simulink model "Copy_of_battery"  (R2021a)
settings: Solver=ode3  StartTime=0.0  StopTime=inf  FixedStep=T_est  RelTol=1e-3  EnableMultiTasking=on
values from neighbouring files (symbols this model uses):
  drive_profile = [0.003069801 0.003247245 0.003020715 0.003053892 0.002820143 0.003317081 0.003158873 0.002919445 0.002956375 0.002698265 0.002861501 0.002770798 ... (18750 elements, 1x18750)]    [drive_profile_ftp.mat]    (also in workspace.mat = [0 0 0 0 0 0 0 0 0 0 0 0 ... (521 elements, 1x521)]; workspace_2rc.mat; workspace_comparison.mat)
  drive_profile_index = [1 2 3 4 5 6 7 8 9 10 11 12 ... (18750 elements, 1x18750)]    [drive_profile_ftp.mat]    (also in load_sim_data_v2.m = drive_profile_index - 1; workspace.mat = [0 0.115384615385 0.230769230769 0.346153846154 0.4615384615; workspace_2rc.mat; workspace_comparison.mat)
  initial_soc = interp1(voc_soc_lut, voc_soc_lut_index, initial_vterm)    [load_sim_data.m]    (also in load_sim_data_v2.m)
  Q_total = 236.8    [load_sim_data.m]    (also in load_sim_data_v2.m = 350; workspace.mat = 44; workspace_2rc.mat = 44; workspace_comparison.mat = 44)
  R1 = interp2(temp_array, voc_array, R1_array, initial_temp, initial_voc)    [load_sim_data.m]    (also in load_sim_data_v2.m; workspace.mat = 0.00033425; workspace_2rc.mat = 0.0001483; workspace_comparison.mat = 0.0001483)
  R2 = interp2(temp_array, voc_array, R2_array, initial_temp, initial_voc)    [load_sim_data.m]    (also in load_sim_data_v2.m; workspace.mat = 0.000915125; workspace_2rc.mat = 0.0001594; workspace_comparison.mat = 0.0001594)
  Ri = interp2(temp_array, voc_array, Ri_array, initial_temp, initial_voc)    [load_sim_data.m]    (also in load_sim_data_v2.m; workspace.mat = 0.000736040625; workspace_2rc.mat = 0.0007932; workspace_comparison.mat = 0.0007932)
  sim_time = drive_profile_index(end)    [load_sim_data.m]    (also in load_sim_data_v2.m)
  voc_soc_lut = [3.07420931 3.44278771 3.51037487 3.58546258 3.63776945 3.68066188 3.73931818 3.84140797 3.94332291 4.0535654 4.18301283]    [emf_curve_single.mat]    (also in workspace.mat = [2.9985 3.0047 3.1504 3.2397 3.3026 3.3438 3.3699 3.3878 3.4; workspace_2rc.mat = [2.9985 3.0047 3.1504 3.2397 3.3026 3.3438 3.3699 3.3878 3.4; workspace_comparison.mat = [2.9985 3.0047 3.1504 3.2397 3.3026 3.3438 3.3699 3.3878 3.4)
  voc_soc_lut_index = [0 10 20 30 40 50 60 70 80 90 100]    [emf_curve_single.mat]    (also in workspace.mat = [0 1.6393442623 3.27868852459 4.91803278689 6.55737704918 8.; workspace_2rc.mat = [0 1.6393442623 3.27868852459 4.91803278689 6.55737704918 8.; workspace_comparison.mat = [0 1.6393442623 3.27868852459 4.91803278689 6.55737704918 8.)
libraries: fl_lib x17, nesl_utility x11
settings Model: Creator=OTG00077  LastModifiedBy=avramkachura
settings SolverCC: AlgebraicLoopSolver=TrustRegion
settings DataIOCC: LimitDataPoints=on  SaveFormat=Array  ReturnWorkspaceOutputs=off
settings OptimizationCC: LifeSpan=inf
settings DebuggingCC: SolverPrmCheckMsg=warning  SFUnexpectedBacktrackingDiag=warning  SFNoUnconditionalDefaultTransitionDiag=warning  SFExecutionAtInitializationDiag=none  SFMachineParentedDataDiag=warning  ArithmeticOperatorsInVariantConditions=warning
settings HardwareCC: ProdBitPerPointer=32  ProdBitPerSizeT=32  ProdBitPerPtrDiffT=32  ProdLargestAtomicFloat=None  ProdIntDivRoundTo=Undefined  ProdEndianess=Unspecified  ProdWordSize=32  ProdHWDeviceType=32-bit Generic
settings ModelReferenceCC: PropagateSignalLabelsOutOfModel=off
settings SFSimCC: SimUseLocalCustomCode=off  CustomCodeUndefinedFunction=UseInterfaceOnly
settings RTWCC: RTWUseLocalCustomCode=off
settings CodeAppCC: StateflowObjectComments=on
settings GRTTargetCC: TargetLangStandard=C89/C90 (ANSI)
settings ConfigComp: CovMetricSettings=dw  CovSaveCumulativeToWorkspaceVar=on  CovSaveSingleToWorkspaceVar=on  CovExternalEMLEnable=off  CovSFcnEnable=off
settings SimscapeCC: SimscapeNormalizeSystem=off

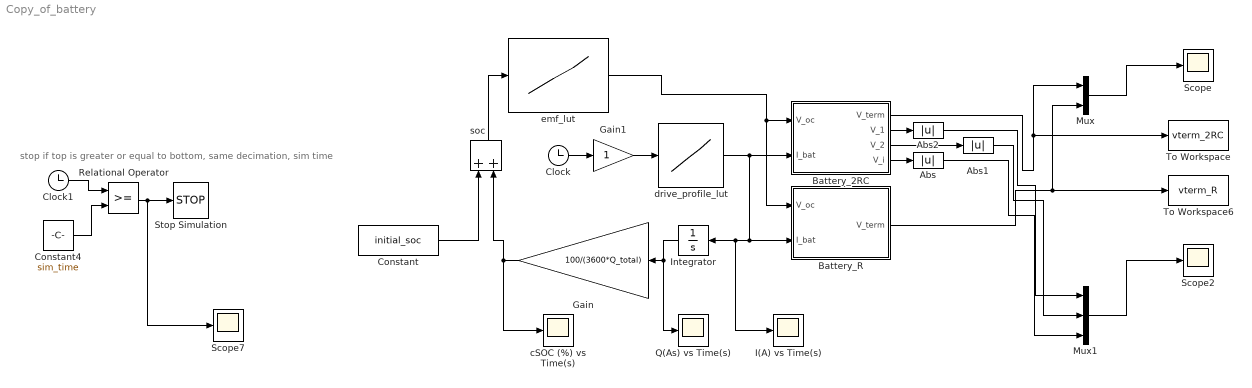
== system Copy_of_battery ==
  note: stop if top is greater or equal to bottom, same decimation, sim time
  Abs : Abs
  Abs1 : Abs
  Abs2 : Abs
  Battery_2RC : Subsystem
  Battery_R : Subsystem
  Clock : Clock
      settings: Decimation=100
  Clock1 : Clock
      settings: Decimation=100
  Constant : Constant  Value=initial_soc
  Constant4 : Constant  Value=sim_time
  Gain : Gain  Gain=100/(3600*Q_total)
  Gain1 : Gain
  I(A) vs Time(s) : Scope
  Integrator : Integrator
  Mux : Mux  Inputs=2
  Mux1 : Mux  Inputs=3
  Q(As) vs Time(s) : Scope
  Relational Operator : RelationalOperator  OutDataTypeStr=boolean  RndMeth=Simplest
  Scope : Scope
  Scope2 : Scope
  Scope7 : Scope
  Stop Simulation : Stop
  To Workspace : ToWorkspace  VariableName=vterm_2RC  SampleTime=-1
      settings: Decimation=100
  To Workspace6 : ToWorkspace  VariableName=vterm_R  SampleTime=-1
      settings: Decimation=100
  "cSOC (%) vs Time(s) " : Scope
  drive_profile_lut : Lookup_n-D  NumberOfTableDimensions=1  BreakpointsForDimension1=drive_profile_index  Table=drive_profile  InternalRulePriority=Speed  RndMeth=Simplest  InputSameDT=on
  emf_lut : Lookup_n-D  NumberOfTableDimensions=1  BreakpointsForDimension1=voc_soc_lut_index  Table=voc_soc_lut  InternalRulePriority=Speed  RndMeth=Simplest  InputSameDT=on
  soc : Sum
  wires:
  Integrator/1 -> Q(As) vs Time(s)/1, Gain/1
  Gain/1 -> "cSOC (%) vs Time(s) "/1, soc/2
  soc/1 -> emf_lut/1
  Constant/1 -> soc/1
  emf_lut/1 -> Battery_R/1(V_oc), Battery_2RC/1(V_oc)
  drive_profile_lut/1 -> Battery_2RC/2(I_bat), I(A) vs Time(s)/1, Integrator/1, Battery_R/2(I_bat)
  Battery_2RC/1(V_term) -> Mux/1, To Workspace/1
  Clock/1 -> Gain1/1
  Gain1/1 -> drive_profile_lut/1
  Mux/1 -> Scope/1
  Battery_R/1(V_term) -> Mux/2, To Workspace6/1
  Battery_2RC/4(V_i) -> Abs/1
  Battery_2RC/3(V_2) -> Abs1/1
  Battery_2RC/2(V_1) -> Abs2/1
  Abs2/1 -> Mux1/1
  Abs1/1 -> Mux1/2
  Abs/1 -> Mux1/3
  Mux1/1 -> Scope2/1
  Relational Operator/1 -> Scope7/1, Stop Simulation/1
  Constant4/1 -> Relational Operator/2
  Clock1/1 -> Relational Operator/1

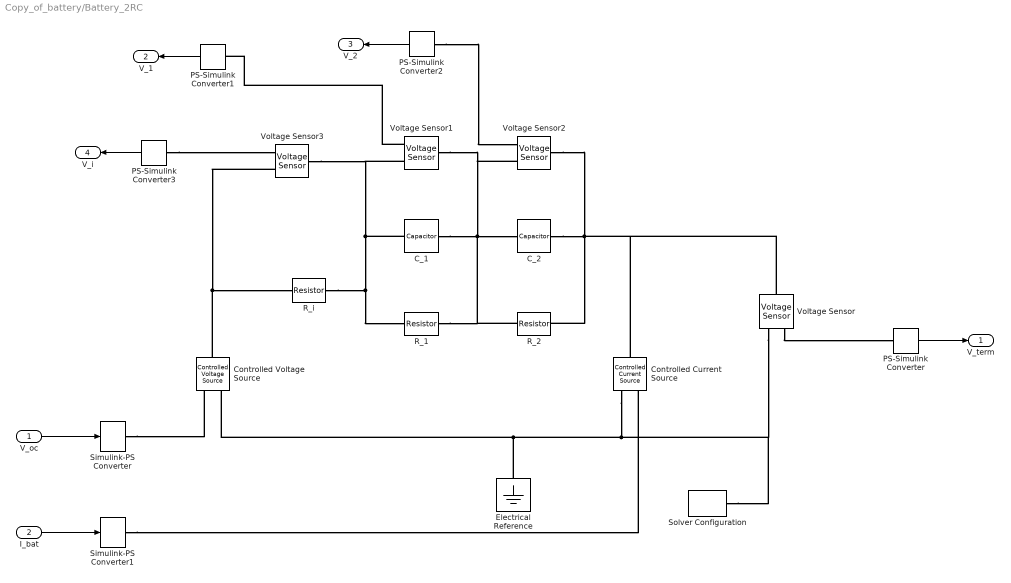
== system Copy_of_battery/Battery_2RC ==
  V_oc : Inport
  I_bat : Inport  Port=2
  C_1 : fl_lib/Electrical/Electrical Elements/Capacitor  c=C1 F  r=0 Ohm  g=0 1/Ohm  i_specify=off  i_priority=High  i=0 A  i_nominal_specify=off  i_nominal_unit=A  i_nominal_value=1  v_specify=off  v_priority=High  v=0 V  v_nominal_specify=off  v_nominal_unit=V  v_nominal_value=1  vc_specify=off  vc_priority=High  vc=0 V  vc_nominal_specify=off  vc_nominal_unit=V  vc_nominal_value=1
  C_2 : fl_lib/Electrical/Electrical Elements/Capacitor  c=C2 F  r=0 Ohm  g=0 1/Ohm  i_specify=off  i_priority=High  i=0 A  i_nominal_specify=off  i_nominal_unit=A  i_nominal_value=1  v_specify=off  v_priority=High  v=0 V  v_nominal_specify=off  v_nominal_unit=V  v_nominal_value=1  vc_specify=off  vc_priority=High  vc=0 V  vc_nominal_specify=off  vc_nominal_unit=V  vc_nominal_value=1
  Controlled Current Source : fl_lib/Electrical/Electrical Sources/Controlled Current Source
  Controlled Voltage Source : fl_lib/Electrical/Electrical Sources/Controlled Voltage Source
  Electrical Reference : fl_lib/Electrical/Electrical Elements/Electrical Reference
  PS-Simulink Converter{,1..3} (4 alike) : nesl_utility/PS-Simulink Converter  PhysicalDomain=network_engine_domain  SubClassName=ps_output  LeftPortType=input  RightPortType=output  PseudoPeriodic=off  Frequencies=[]  Unit=1  AffineConversion=off
      settings: SourceProductBaseCode=PW,SS
  R_1 : fl_lib/Electrical/Electrical Elements/Resistor  R=R1 Ohm  i_specify=off  i_priority=High  i=0 A  i_nominal_specify=off  i_nominal_unit=A  i_nominal_value=1  v_specify=off  v_priority=High  v=0 V  v_nominal_specify=off  v_nominal_unit=V  v_nominal_value=1
  R_2 : fl_lib/Electrical/Electrical Elements/Resistor  R=R2 Ohm  i_specify=off  i_priority=High  i=0 A  i_nominal_specify=off  i_nominal_unit=A  i_nominal_value=1  v_specify=off  v_priority=High  v=0 V  v_nominal_specify=off  v_nominal_unit=V  v_nominal_value=1
  R_i : fl_lib/Electrical/Electrical Elements/Resistor  R=Ri Ohm  i_specify=off  i_priority=High  i=0 A  i_nominal_specify=off  i_nominal_unit=A  i_nominal_value=1  v_specify=off  v_priority=High  v=0 V  v_nominal_specify=off  v_nominal_unit=V  v_nominal_value=1
  Simulink-PS Converter : nesl_utility/Simulink-PS Converter  PhysicalDomain=network_engine_domain  SubClassName=ps_input  LeftPortType=input  RightPortType=output  PseudoPeriodic=off  Frequencies=[]  NoiseDistribution=none  NoiseParameters=[]  Unit=1  AffineConversion=off  FilteringAndDerivatives=zero  SimscapeFilterOrder=1  InputFilterTimeConstant=0.001  UdotUserProvided=1
      settings: SourceProductBaseCode=PW,SS
  Simulink-PS Converter1 : nesl_utility/Simulink-PS Converter  PhysicalDomain=network_engine_domain  SubClassName=ps_input  LeftPortType=input  RightPortType=output  PseudoPeriodic=off  Frequencies=[]  NoiseDistribution=none  NoiseParameters=[]  Unit=1  AffineConversion=off  FilteringAndDerivatives=zero  SimscapeFilterOrder=1  InputFilterTimeConstant=0.001  UdotUserProvided=1
      settings: SourceProductBaseCode=PW,SS
  Solver Configuration : nesl_utility/Solver Configuration  PhysicalDomain=network_engine_domain  SubClassName=solver  LeftPortType=input  RightPortType=generic  Tones=[]  Harmonics=[]  SimulateNoise=off  Profile=off  UseLocalSampling=off  EnableSwitchedLinearOptims=on  FrequencyDomain=off  UseCCode=off  RelTol=0.001  AbsTol=1e-06  MinStep=1e-09  ToWorkspace=off  RevertToSquareIcSolve=off  NumHomotopyIterations=100  PhasorMode=off  PhasorModeNumHarmonics=1  DoDC=off  ResidualTolerance=1e-09  UseLocalSolver=off  LocalSolverChoice=NE_BACKWARD_EULER_ADVANCER  LocalSolverSampleTime=0.001  DoFixedCost=off  MaxNonlinIter=3  MaxModeIter=2  ComputeImpulses=off  ImpulseIterations=2  LinearAlgebra=Sparse  EquationFormulation=NE_TIME_EF  DelaysMemoryBudget=1024  AutomaticFiltering=on  FilteringTimeConstant=0.001  PartitionStorageMethod=AS_NEEDED  PartitionMemoryBudget=1024  PartitionMethod=FAST
      settings: SourceProductBaseCode=PW,SS
  Voltage Sensor{,1..3} (4 alike) : fl_lib/Electrical/Electrical Sensors/Voltage Sensor
  V_term : Outport  VectorParamsAs1DForOutWhenUnconnected=off
  V_1 : Outport  Port=2  VectorParamsAs1DForOutWhenUnconnected=off
  V_2 : Outport  Port=3  VectorParamsAs1DForOutWhenUnconnected=off
  V_i : Outport  Port=4  VectorParamsAs1DForOutWhenUnconnected=off
  wires:
  V_oc/1 -> Simulink-PS Converter/1
  PS-Simulink Converter/1 -> V_term/1
  I_bat/1 -> Simulink-PS Converter1/1
  PS-Simulink Converter1/1 -> V_1/1
  PS-Simulink Converter2/1 -> V_2/1
  PS-Simulink Converter3/1 -> V_i/1
  connections:
  R_i/RConn1 -- Voltage Sensor3/LConn1 -- Voltage Sensor1/RConn2 -- C_1/LConn1 -- R_1/LConn1
  C_1/RConn1 -- Voltage Sensor2/RConn2 -- Voltage Sensor1/LConn1 -- R_2/LConn1 -- R_1/RConn1 -- C_2/LConn1
  C_2/RConn1 -- Voltage Sensor2/LConn1 -- R_2/RConn1 -- Controlled Current Source/LConn1 -- Voltage Sensor/LConn1
  Controlled Voltage Source/LConn1 -- Voltage Sensor3/RConn2 -- R_i/LConn1
  Simulink-PS Converter/RConn1 -- Controlled Voltage Source/RConn1
  Voltage Sensor/RConn1 -- PS-Simulink Converter/LConn1
  Controlled Current Source/RConn2 -- Solver Configuration/RConn1 -- Voltage Sensor/RConn2 -- Electrical Reference/LConn1 -- Controlled Voltage Source/RConn2
  Simulink-PS Converter1/RConn1 -- Controlled Current Source/RConn1
  Voltage Sensor1/RConn1 -- PS-Simulink Converter1/LConn1
  PS-Simulink Converter2/LConn1 -- Voltage Sensor2/RConn1
  PS-Simulink Converter3/LConn1 -- Voltage Sensor3/RConn1

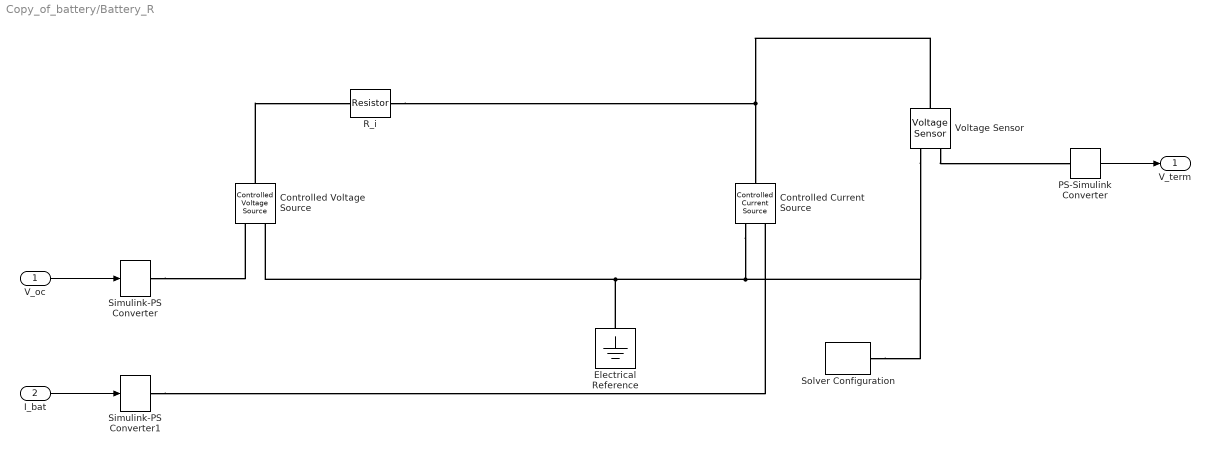
== system Copy_of_battery/Battery_R ==
  V_oc : Inport
  I_bat : Inport  Port=2
  Controlled Current Source : fl_lib/Electrical/Electrical Sources/Controlled Current Source
  Controlled Voltage Source : fl_lib/Electrical/Electrical Sources/Controlled Voltage Source
  Electrical Reference : fl_lib/Electrical/Electrical Elements/Electrical Reference
  PS-Simulink Converter : nesl_utility/PS-Simulink Converter  PhysicalDomain=network_engine_domain  SubClassName=ps_output  LeftPortType=input  RightPortType=output  PseudoPeriodic=off  Frequencies=[]  Unit=1  AffineConversion=off
      settings: SourceProductBaseCode=PW,SS
  R_i : fl_lib/Electrical/Electrical Elements/Resistor  R=Ri+R1+R2 Ohm  i_specify=off  i_priority=High  i=0 A  i_nominal_specify=off  i_nominal_unit=A  i_nominal_value=1  v_specify=off  v_priority=High  v=0 V  v_nominal_specify=off  v_nominal_unit=V  v_nominal_value=1
  Simulink-PS Converter : nesl_utility/Simulink-PS Converter  PhysicalDomain=network_engine_domain  SubClassName=ps_input  LeftPortType=input  RightPortType=output  PseudoPeriodic=off  Frequencies=[]  NoiseDistribution=none  NoiseParameters=[]  Unit=1  AffineConversion=off  FilteringAndDerivatives=zero  SimscapeFilterOrder=1  InputFilterTimeConstant=0.001  UdotUserProvided=1
      settings: SourceProductBaseCode=PW,SS
  Simulink-PS Converter1 : nesl_utility/Simulink-PS Converter  PhysicalDomain=network_engine_domain  SubClassName=ps_input  LeftPortType=input  RightPortType=output  PseudoPeriodic=off  Frequencies=[]  NoiseDistribution=none  NoiseParameters=[]  Unit=1  AffineConversion=off  FilteringAndDerivatives=zero  SimscapeFilterOrder=1  InputFilterTimeConstant=0.001  UdotUserProvided=1
      settings: SourceProductBaseCode=PW,SS
  Solver Configuration : nesl_utility/Solver Configuration  PhysicalDomain=network_engine_domain  SubClassName=solver  LeftPortType=input  RightPortType=generic  Tones=[]  Harmonics=[]  SimulateNoise=off  Profile=off  UseLocalSampling=off  EnableSwitchedLinearOptims=on  FrequencyDomain=off  UseCCode=off  RelTol=0.001  AbsTol=1e-06  MinStep=1e-09  ToWorkspace=off  RevertToSquareIcSolve=off  NumHomotopyIterations=100  PhasorMode=off  PhasorModeNumHarmonics=1  DoDC=off  ResidualTolerance=1e-09  UseLocalSolver=off  LocalSolverChoice=NE_BACKWARD_EULER_ADVANCER  LocalSolverSampleTime=0.001  DoFixedCost=off  MaxNonlinIter=3  MaxModeIter=2  ComputeImpulses=off  ImpulseIterations=2  LinearAlgebra=Sparse  EquationFormulation=NE_TIME_EF  DelaysMemoryBudget=1024  AutomaticFiltering=on  FilteringTimeConstant=0.001  PartitionStorageMethod=AS_NEEDED  PartitionMemoryBudget=1024  PartitionMethod=FAST
      settings: SourceProductBaseCode=PW,SS
  Voltage Sensor : fl_lib/Electrical/Electrical Sensors/Voltage Sensor
  V_term : Outport  VectorParamsAs1DForOutWhenUnconnected=off
  wires:
  V_oc/1 -> Simulink-PS Converter/1
  PS-Simulink Converter/1 -> V_term/1
  I_bat/1 -> Simulink-PS Converter1/1
  connections:
  Voltage Sensor/LConn1 -- Controlled Current Source/LConn1 -- R_i/RConn1
  Controlled Voltage Source/LConn1 -- R_i/LConn1
  Simulink-PS Converter/RConn1 -- Controlled Voltage Source/RConn1
  Voltage Sensor/RConn1 -- PS-Simulink Converter/LConn1
  Controlled Current Source/RConn2 -- Solver Configuration/RConn1 -- Voltage Sensor/RConn2 -- Electrical Reference/LConn1 -- Controlled Voltage Source/RConn2
  Simulink-PS Converter1/RConn1 -- Controlled Current Source/RConn1
